simulink library "halin"  (R2021b)
settings: Solver=VariableStepAuto  StartTime=0.0  StopTime=10.0  RelTol=1e-3
undefined symbols (not defined in the file): TRUE
libraries: FVT_lib x177, hcu_lib x55
(part 4 of 17)

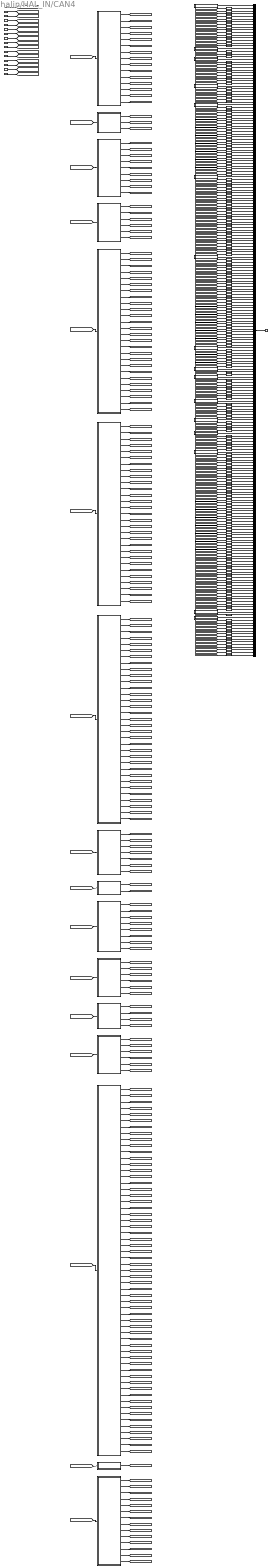
== system halin/HAL_IN/CAN4 ==
  DT_CAN4_SG_DKC1 : Inport
  DT_CAN4_SG_DKC2 : Inport  Port=2
  DT_CAN4_SG_PTG1 : Inport  Port=3
  DT_CAN4_SG_ZONE_DR1 : Inport  Port=4
  DT_CAN4_SG_ZONE_DR_VCU : Inport  Port=5
  DT_CAN4_SG_ZONE_FR1 : Inport  Port=6
  DT_CAN4_SG_ZONE_FR_VCU : Inport  Port=7
  DT_CAN4_SG_ZONE_L1 : Inport  Port=8
  DT_CAN4_SG_ZONE_L2 : Inport  Port=9
  DT_CAN4_SG_ZONE_R1 : Inport  Port=10
  DT_CAN4_SG_ZONE_R2 : Inport  Port=11
  DT_CAN4_SG_zGW_APTC1 : Inport  Port=12
  DT_CAN4_SG_zGW_CANFr1 : Inport  Port=13
  DT_CAN4_SG_zGW_LINDr1 : Inport  Port=14
  DT_CAN4_SG_zGW_LINFr1 : Inport  Port=15
  DT_CAN4_SG_zGW_SEAT1 : Inport  Port=16
  DKC1 : Subsystem
  DKC2 : Subsystem
  PTG1 : Subsystem
  UnitConverter{,1..11,13,18,21..22,24..26,33,39,41,43,45,47,49,51,53,55,57..58,82,88,90,92..97,100,102,104,106,108,110,112,114..118,120,124..127,131..134,137,140..143,155..156,158..160,165,169,173,177,180,213,218,220..221,224,226..227} (83 alike) : DataTypeConversion  OutDataTypeStr=uint8
  UnitConverter{29..30,38,40,42,44,46,48,50,52,54,56,61,63,84..87,89,91,99,101,103,105,107,109,111,113,119,128..129,138..139,144..152,164,168,172,176} (46 alike) : DataTypeConversion  OutDataTypeStr=single
  UnitConverter{12,14,19..20,23,27..28,31..32,34..37,59..60,62,64..81,83,98,121..123,130,135..136,154,157,161..163,166..167,170..171,174..175,178..179,181..212,214..216,222} (91 alike) : DataTypeConversion  OutDataTypeStr=boolean
  UnitConverter15 : DataTypeConversion  OutDataTypeStr=uint64
  UnitConverter{153,217,219,223,225} (5 alike) : DataTypeConversion  OutDataTypeStr=uint16
  UnitConverter16 : DataTypeConversion  OutDataTypeStr=uint64
  UnitConverter17 : DataTypeConversion  OutDataTypeStr=uint64
  VHAL_CANMsgInvalidDKC1_flg : Subsystem  AncestorBlock=FVT_lib/hal/MsgTimeoutJudge_CAN_AUTOSAR
      mask help: MeasumentTrigerEvent
      mask Display: fprintf('MsgTimeoutJudge_CAN\nAUTOSAR');
  VHAL_CANMsgInvalidDKC2_flg : Subsystem  AncestorBlock=FVT_lib/hal/MsgTimeoutJudge_CAN_AUTOSAR
      mask help: MeasumentTrigerEvent
      mask Display: fprintf('MsgTimeoutJudge_CAN\nAUTOSAR');
  VHAL_CANMsgInvalidPTG1_flg : Subsystem  AncestorBlock=FVT_lib/hal/MsgTimeoutJudge_CAN_AUTOSAR
      mask help: MeasumentTrigerEvent
      mask Display: fprintf('MsgTimeoutJudge_CAN\nAUTOSAR');
  VHAL_CANMsgInvalidZONEDR1_flg : Subsystem  AncestorBlock=FVT_lib/hal/MsgTimeoutJudge_CAN_AUTOSAR
      mask help: MeasumentTrigerEvent
      mask Display: fprintf('MsgTimeoutJudge_CAN\nAUTOSAR');
  VHAL_CANMsgInvalidZONEDRVCU_flg : Subsystem  AncestorBlock=FVT_lib/hal/MsgTimeoutJudge_CAN_AUTOSAR
      mask help: MeasumentTrigerEvent
      mask Display: fprintf('MsgTimeoutJudge_CAN\nAUTOSAR');
  VHAL_CANMsgInvalidZONEFR1_flg : Subsystem  AncestorBlock=FVT_lib/hal/MsgTimeoutJudge_CAN_AUTOSAR
      mask help: MeasumentTrigerEvent
      mask Display: fprintf('MsgTimeoutJudge_CAN\nAUTOSAR');
  VHAL_CANMsgInvalidZONEFRVCU_flg : Subsystem  AncestorBlock=FVT_lib/hal/MsgTimeoutJudge_CAN_AUTOSAR
      mask help: MeasumentTrigerEvent
      mask Display: fprintf('MsgTimeoutJudge_CAN\nAUTOSAR');
  VHAL_CANMsgInvalidZONEL1_flg : Subsystem  AncestorBlock=FVT_lib/hal/MsgTimeoutJudge_CAN_AUTOSAR
      mask help: MeasumentTrigerEvent
      mask Display: fprintf('MsgTimeoutJudge_CAN\nAUTOSAR');
  VHAL_CANMsgInvalidZONEL2_flg : Subsystem  AncestorBlock=FVT_lib/hal/MsgTimeoutJudge_CAN_AUTOSAR
      mask help: MeasumentTrigerEvent
      mask Display: fprintf('MsgTimeoutJudge_CAN\nAUTOSAR');
  VHAL_CANMsgInvalidZONER1_flg : Subsystem  AncestorBlock=FVT_lib/hal/MsgTimeoutJudge_CAN_AUTOSAR
      mask help: MeasumentTrigerEvent
      mask Display: fprintf('MsgTimeoutJudge_CAN\nAUTOSAR');
  VHAL_CANMsgInvalidZONER2_flg : Subsystem  AncestorBlock=FVT_lib/hal/MsgTimeoutJudge_CAN_AUTOSAR
      mask help: MeasumentTrigerEvent
      mask Display: fprintf('MsgTimeoutJudge_CAN\nAUTOSAR');
  VHAL_CANMsgInvalidzGWAPTC1_flg : Subsystem  AncestorBlock=FVT_lib/hal/MsgTimeoutJudge_CAN_AUTOSAR
      mask help: MeasumentTrigerEvent
      mask Display: fprintf('MsgTimeoutJudge_CAN\nAUTOSAR');
  VHAL_CANMsgInvalidzGWCANFr1_flg : Subsystem  AncestorBlock=FVT_lib/hal/MsgTimeoutJudge_CAN_AUTOSAR
      mask help: MeasumentTrigerEvent
      mask Display: fprintf('MsgTimeoutJudge_CAN\nAUTOSAR');
  VHAL_CANMsgInvalidzGWLINDr1_flg : Subsystem  AncestorBlock=FVT_lib/hal/MsgTimeoutJudge_CAN_AUTOSAR
      mask help: MeasumentTrigerEvent
      mask Display: fprintf('MsgTimeoutJudge_CAN\nAUTOSAR');
  VHAL_CANMsgInvalidzGWLINFr1_flg : Subsystem  AncestorBlock=FVT_lib/hal/MsgTimeoutJudge_CAN_AUTOSAR
      mask help: MeasumentTrigerEvent
      mask Display: fprintf('MsgTimeoutJudge_CAN\nAUTOSAR');
  VHAL_CANMsgInvalidzGWSEAT1_flg : Subsystem  AncestorBlock=FVT_lib/hal/MsgTimeoutJudge_CAN_AUTOSAR
      mask help: MeasumentTrigerEvent
      mask Display: fprintf('MsgTimeoutJudge_CAN\nAUTOSAR');
  ZONE_DR1 : Subsystem
  ZONE_DR_VCU : Subsystem
  ZONE_FR1 : Subsystem
  ZONE_FR_VCU : Subsystem
  ZONE_L1 : Subsystem
  ZONE_L2 : Subsystem
  ZONE_R1 : Subsystem
  ZONE_R2 : Subsystem
  bus_creator : BusCreator  Inputs=244
  zGW_APTC1 : Subsystem
  zGW_CANFr1 : Subsystem
  zGW_LINDr1 : Subsystem
  zGW_LINFr1 : Subsystem
  zGW_SEAT1 : Subsystem
  HAL_CAN4_outputs : Outport
  wires:
  DT_CAN4_SG_DKC1/1 -> [DT_CAN4_SG_DKC1]
  DT_CAN4_SG_DKC2/1 -> [DT_CAN4_SG_DKC2]
  DT_CAN4_SG_PTG1/1 -> [DT_CAN4_SG_PTG1]
  DT_CAN4_SG_ZONE_DR1/1 -> [DT_CAN4_SG_ZONE_DR1]
  DT_CAN4_SG_ZONE_DR_VCU/1 -> [DT_CAN4_SG_ZONE_DR_VCU]
  DT_CAN4_SG_ZONE_FR1/1 -> [DT_CAN4_SG_ZONE_FR1]
  DT_CAN4_SG_ZONE_FR_VCU/1 -> [DT_CAN4_SG_ZONE_FR_VCU]
  DT_CAN4_SG_ZONE_L1/1 -> [DT_CAN4_SG_ZONE_L1]
  DT_CAN4_SG_ZONE_L2/1 -> [DT_CAN4_SG_ZONE_L2]
  DT_CAN4_SG_ZONE_R1/1 -> [DT_CAN4_SG_ZONE_R1]
  DT_CAN4_SG_ZONE_R2/1 -> [DT_CAN4_SG_ZONE_R2]
  DT_CAN4_SG_zGW_APTC1/1 -> [DT_CAN4_SG_zGW_APTC1]
  DT_CAN4_SG_zGW_CANFr1/1 -> [DT_CAN4_SG_zGW_CANFr1]
  DT_CAN4_SG_zGW_LINDr1/1 -> [DT_CAN4_SG_zGW_LINDr1]
  DT_CAN4_SG_zGW_LINFr1/1 -> [DT_CAN4_SG_zGW_LINFr1]
  DT_CAN4_SG_zGW_SEAT1/1 -> [DT_CAN4_SG_zGW_SEAT1]
  [DT_CAN4_SG_DKC1] -> DKC1/1(DT_CAN4_SG_DKC1)
  [DT_CAN4_SG_DKC2] -> DKC2/1(DT_CAN4_SG_DKC2)
  [DT_CAN4_SG_PTG1] -> PTG1/1(DT_CAN4_SG_PTG1)
  [DT_CAN4_SG_ZONE_DR1] -> ZONE_DR1/1(DT_CAN4_SG_ZONE_DR1)
  [DT_CAN4_SG_ZONE_DR_VCU] -> ZONE_DR_VCU/1(DT_CAN4_SG_ZONE_DR_VCU)
  [DT_CAN4_SG_ZONE_FR1] -> ZONE_FR1/1(DT_CAN4_SG_ZONE_FR1)
  [DT_CAN4_SG_ZONE_FR_VCU] -> ZONE_FR_VCU/1(DT_CAN4_SG_ZONE_FR_VCU)
  [DT_CAN4_SG_ZONE_L1] -> ZONE_L1/1(DT_CAN4_SG_ZONE_L1)
  [DT_CAN4_SG_ZONE_L2] -> ZONE_L2/1(DT_CAN4_SG_ZONE_L2)
  [DT_CAN4_SG_ZONE_R1] -> ZONE_R1/1(DT_CAN4_SG_ZONE_R1)
  [DT_CAN4_SG_ZONE_R2] -> ZONE_R2/1(DT_CAN4_SG_ZONE_R2)
  [DT_CAN4_SG_zGW_APTC1] -> zGW_APTC1/1(DT_CAN4_SG_zGW_APTC1)
  [DT_CAN4_SG_zGW_CANFr1] -> zGW_CANFr1/1(DT_CAN4_SG_zGW_CANFr1)
  [DT_CAN4_SG_zGW_LINDr1] -> zGW_LINDr1/1(DT_CAN4_SG_zGW_LINDr1)
  [DT_CAN4_SG_zGW_LINFr1] -> zGW_LINFr1/1(DT_CAN4_SG_zGW_LINFr1)
  [DT_CAN4_SG_zGW_SEAT1] -> zGW_SEAT1/1(DT_CAN4_SG_zGW_SEAT1)
  bus_creator/1 -> HAL_CAN4_outputs/1
  VHAL_CANMsgInvalidDKC1_flg/1(Out) -> bus_creator/1
  DKC1/1(VHAL_DKCKeyNumSta_enum) -> [VHAL_DKCKeyNumSta_enum]
  UnitConverter/1 -> bus_creator/2  "VHAL_DKCKeyNumSta_enum"
  [VHAL_DKCKeyNumSta_enum] -> UnitConverter/1
  DKC1/2(VHAL_DKCKeyTypeSta_enum) -> [VHAL_DKCKeyTypeSta_enum]
  UnitConverter1/1 -> bus_creator/3  "VHAL_DKCKeyTypeSta_enum"
  [VHAL_DKCKeyTypeSta_enum] -> UnitConverter1/1
  DKC1/3(VHAL_DKCPDkeyAreaRAPSSta_enum) -> [VHAL_DKCPDkeyAreaRAPSSta_enum]
  UnitConverter2/1 -> bus_creator/4  "VHAL_DKCPDkeyAreaRAPSSta_enum"
  [VHAL_DKCPDkeyAreaRAPSSta_enum] -> UnitConverter2/1
  DKC1/4(VHAL_DKCParkingModeCmd_enum) -> [VHAL_DKCParkingModeCmd_enum]
  UnitConverter3/1 -> bus_creator/5  "VHAL_DKCParkingModeCmd_enum"
  [VHAL_DKCParkingModeCmd_enum] -> UnitConverter3/1
  DKC1/5(VHAL_DKCReVehData_enum) -> [VHAL_DKCReVehData_enum]
  UnitConverter4/1 -> bus_creator/6  "VHAL_DKCReVehData_enum"
  [VHAL_DKCReVehData_enum] -> UnitConverter4/1
  DKC1/6(VHAL_PCommandToBCM_enum) -> [VHAL_PCommandToBCM_enum]
  UnitConverter5/1 -> bus_creator/7  "VHAL_PCommandToBCM_enum"
  [VHAL_PCommandToBCM_enum] -> UnitConverter5/1
  DKC1/7(VHAL_PCommandToPTG_enum) -> [VHAL_PCommandToPTG_enum]
  UnitConverter6/1 -> bus_creator/8  "VHAL_PCommandToPTG_enum"
  [VHAL_PCommandToPTG_enum] -> UnitConverter6/1
  DKC1/8(VHAL_PDKeyAreaLockUnlock_enum) -> [VHAL_PDKeyAreaLockUnlock_enum]
  UnitConverter7/1 -> bus_creator/9  "VHAL_PDKeyAreaLockUnlock_enum"
  [VHAL_PDKeyAreaLockUnlock_enum] -> UnitConverter7/1
  DKC1/9(VHAL_PDKeyAreaPS_enum) -> [VHAL_PDKeyAreaPS_enum]
  UnitConverter8/1 -> bus_creator/10  "VHAL_PDKeyAreaPS_enum"
  [VHAL_PDKeyAreaPS_enum] -> UnitConverter8/1
  DKC1/10(VHAL_PDKeyAreaPTG_enum) -> [VHAL_PDKeyAreaPTG_enum]
  UnitConverter9/1 -> bus_creator/11  "VHAL_PDKeyAreaPTG_enum"
  [VHAL_PDKeyAreaPTG_enum] -> UnitConverter9/1
  DKC1/11(VHAL_PDKeyWelcome_enum) -> [VHAL_PDKeyWelcome_enum]
  UnitConverter10/1 -> bus_creator/12  "VHAL_PDKeyWelcome_enum"
  [VHAL_PDKeyWelcome_enum] -> UnitConverter10/1
  DKC1/12(VHAL_PDkeyShowIVI_enum) -> [VHAL_PDkeyShowIVI_enum]
  UnitConverter11/1 -> bus_creator/13  "VHAL_PDkeyShowIVI_enum"
  [VHAL_PDkeyShowIVI_enum] -> UnitConverter11/1
  DKC1/13(VHAL_PKeyMiss_flg) -> [VHAL_PKeyMiss_flg]
  UnitConverter12/1 -> bus_creator/14  "VHAL_PKeyMiss_flg"
  [VHAL_PKeyMiss_flg] -> UnitConverter12/1
  DKC1/14(VHAL_PKeyMode_enum) -> [VHAL_PKeyMode_enum]
  UnitConverter13/1 -> bus_creator/15  "VHAL_PKeyMode_enum"
  [VHAL_PKeyMode_enum] -> UnitConverter13/1
  DKC1/15(VHAL_PUIDLowPower_flg) -> [VHAL_PUIDLowPower_flg]
  UnitConverter14/1 -> bus_creator/16  "VHAL_PUIDLowPower_flg"
  [VHAL_PUIDLowPower_flg] -> UnitConverter14/1
  VHAL_CANMsgInvalidDKC2_flg/1(Out) -> bus_creator/17
  DKC2/1(VHAL_EncryptionDATA063_enum) -> [VHAL_EncryptionDATA063_enum]
  UnitConverter15/1 -> bus_creator/18  "VHAL_EncryptionDATA063_enum"
  [VHAL_EncryptionDATA063_enum] -> UnitConverter15/1
  DKC2/2(VHAL_EncryptionDATA64127_enum) -> [VHAL_EncryptionDATA64127_enum]
  UnitConverter16/1 -> bus_creator/19  "VHAL_EncryptionDATA64127_enum"
  [VHAL_EncryptionDATA64127_enum] -> UnitConverter16/1
  DKC2/3(VHAL_RandomNumberX_enum) -> [VHAL_RandomNumberX_enum]
  UnitConverter17/1 -> bus_creator/20  "VHAL_RandomNumberX_enum"
  [VHAL_RandomNumberX_enum] -> UnitConverter17/1
  VHAL_CANMsgInvalidPTG1_flg/1(Out) -> bus_creator/21
  PTG1/1(VHAL_PTGActiveSta_enum) -> [VHAL_PTGActiveSta_enum]
  UnitConverter18/1 -> bus_creator/22  "VHAL_PTGActiveSta_enum"
  [VHAL_PTGActiveSta_enum] -> UnitConverter18/1
  PTG1/2(VHAL_PTGAutoStaus_flg) -> [VHAL_PTGAutoStaus_flg]
  UnitConverter19/1 -> bus_creator/23  "VHAL_PTGAutoStaus_flg"
  [VHAL_PTGAutoStaus_flg] -> UnitConverter19/1
  PTG1/3(VHAL_PTGExist_flg) -> [VHAL_PTGExist_flg]
  UnitConverter20/1 -> bus_creator/24  "VHAL_PTGExist_flg"
  [VHAL_PTGExist_flg] -> UnitConverter20/1
  PTG1/4(VHAL_PTGHWVer_enum) -> [VHAL_PTGHWVer_enum]
  UnitConverter21/1 -> bus_creator/25  "VHAL_PTGHWVer_enum"
  [VHAL_PTGHWVer_enum] -> UnitConverter21/1
  PTG1/5(VHAL_PTGInnerSW2_enum) -> [VHAL_PTGInnerSW2_enum]
  UnitConverter22/1 -> bus_creator/26  "VHAL_PTGInnerSW2_enum"
  [VHAL_PTGInnerSW2_enum] -> UnitConverter22/1
  PTG1/6(VHAL_PTGIsSetHeight_flg) -> [VHAL_PTGIsSetHeight_flg]
  UnitConverter23/1 -> bus_creator/27  "VHAL_PTGIsSetHeight_flg"
  [VHAL_PTGIsSetHeight_flg] -> UnitConverter23/1
  PTG1/7(VHAL_PTGRDILSta_enum) -> [VHAL_PTGRDILSta_enum]
  UnitConverter24/1 -> bus_creator/28  "VHAL_PTGRDILSta_enum"
  [VHAL_PTGRDILSta_enum] -> UnitConverter24/1
  PTG1/8(VHAL_PTGSWVer_enum) -> [VHAL_PTGSWVer_enum]
  UnitConverter25/1 -> bus_creator/29  "VHAL_PTGSWVer_enum"
  [VHAL_PTGSWVer_enum] -> UnitConverter25/1
  PTG1/9(VHAL_PTGSysSta_enum) -> [VHAL_PTGSysSta_enum]
  UnitConverter26/1 -> bus_creator/30  "VHAL_PTGSysSta_enum"
  [VHAL_PTGSysSta_enum] -> UnitConverter26/1
  VHAL_CANMsgInvalidZONEDR1_flg/1(Out) -> bus_creator/31
  ZONE_DR1/1(VHAL_DrLockSta_flg) -> [VHAL_DrLockSta_flg]
  UnitConverter27/1 -> bus_creator/32  "VHAL_DrLockSta_flg"
  [VHAL_DrLockSta_flg] -> UnitConverter27/1
  ZONE_DR1/2(VHAL_MIRRORFOLDSW_flg) -> [VHAL_MIRRORFOLDSW_flg]
  UnitConverter28/1 -> bus_creator/33  "VHAL_MIRRORFOLDSW_flg"
  [VHAL_MIRRORFOLDSW_flg] -> UnitConverter28/1
  ZONE_DR1/3(VHAL_RLTurnLampC_mA) -> [VHAL_RLTurnLampC_mA]
  UnitConverter29/1 -> bus_creator/34  "VHAL_RLTurnLampC_mA"
  [VHAL_RLTurnLampC_mA] -> UnitConverter29/1
  ZONE_DR1/4(VHAL_RRTurnLampC_mA) -> [VHAL_RRTurnLampC_mA]
  UnitConverter30/1 -> bus_creator/35  "VHAL_RRTurnLampC_mA"
  [VHAL_RRTurnLampC_mA] -> UnitConverter30/1
  ZONE_DR1/5(VHAL_RWiperAS_flg) -> [VHAL_RWiperAS_flg]
  UnitConverter31/1 -> bus_creator/36  "VHAL_RWiperAS_flg"
  [VHAL_RWiperAS_flg] -> UnitConverter31/1
  ZONE_DR1/6(VHAL_RWiperProtection_flg) -> [VHAL_RWiperProtection_flg]
  UnitConverter32/1 -> bus_creator/37  "VHAL_RWiperProtection_flg"
  [VHAL_RWiperProtection_flg] -> UnitConverter32/1
  VHAL_CANMsgInvalidZONEDRVCU_flg/1(Out) -> bus_creator/38
  ZONE_DR_VCU/1(VHAL_BlowerErr_enum) -> [VHAL_BlowerErr_enum]
  UnitConverter33/1 -> bus_creator/39  "VHAL_BlowerErr_enum"
  [VHAL_BlowerErr_enum] -> UnitConverter33/1
  ZONE_DR_VCU/2(VHAL_DrPMMLVOutPErrLmp_flg) -> [VHAL_DrPMMLVOutPErrLmp_flg]
  UnitConverter34/1 -> bus_creator/40  "VHAL_DrPMMLVOutPErrLmp_flg"
  [VHAL_DrPMMLVOutPErrLmp_flg] -> UnitConverter34/1
  ZONE_DR_VCU/3(VHAL_DrPMMSysErrLmp_flg) -> [VHAL_DrPMMSysErrLmp_flg]
  UnitConverter35/1 -> bus_creator/41  "VHAL_DrPMMSysErrLmp_flg"
  [VHAL_DrPMMSysErrLmp_flg] -> UnitConverter35/1
  ZONE_DR_VCU/4(VHAL_DrSCPSysErrLmp_flg) -> [VHAL_DrSCPSysErrLmp_flg]
  UnitConverter36/1 -> bus_creator/42  "VHAL_DrSCPSysErrLmp_flg"
  [VHAL_DrSCPSysErrLmp_flg] -> UnitConverter36/1
  ZONE_DR_VCU/5(VHAL_DrStdAErrSta_flg) -> [VHAL_DrStdAErrSta_flg]
  UnitConverter37/1 -> bus_creator/43  "VHAL_DrStdAErrSta_flg"
  [VHAL_DrStdAErrSta_flg] -> UnitConverter37/1
  ZONE_DR_VCU/6(VHAL_SolarL_W) -> [VHAL_SolarL_W]
  UnitConverter38/1 -> bus_creator/44  "VHAL_SolarL_W"
  [VHAL_SolarL_W] -> UnitConverter38/1
  ZONE_DR_VCU/7(VHAL_SolarLErr_enum) -> [VHAL_SolarLErr_enum]
  UnitConverter39/1 -> bus_creator/45  "VHAL_SolarLErr_enum"
  [VHAL_SolarLErr_enum] -> UnitConverter39/1
  ZONE_DR_VCU/8(VHAL_SolarR_W) -> [VHAL_SolarR_W]
  UnitConverter40/1 -> bus_creator/46  "VHAL_SolarR_W"
  [VHAL_SolarR_W] -> UnitConverter40/1
  ZONE_DR_VCU/9(VHAL_SolarRErr_enum) -> [VHAL_SolarRErr_enum]
  UnitConverter41/1 -> bus_creator/47  "VHAL_SolarRErr_enum"
  [VHAL_SolarRErr_enum] -> UnitConverter41/1
  ZONE_DR_VCU/10(VHAL_TFaceL_C) -> [VHAL_TFaceL_C]
  UnitConverter42/1 -> bus_creator/48  "VHAL_TFaceL_C"
  [VHAL_TFaceL_C] -> UnitConverter42/1
  ZONE_DR_VCU/11(VHAL_TFaceLErr_enum) -> [VHAL_TFaceLErr_enum]
  UnitConverter43/1 -> bus_creator/49  "VHAL_TFaceLErr_enum"
  [VHAL_TFaceLErr_enum] -> UnitConverter43/1
  ZONE_DR_VCU/12(VHAL_TFaceR_C) -> [VHAL_TFaceR_C]
  UnitConverter44/1 -> bus_creator/50  "VHAL_TFaceR_C"
  [VHAL_TFaceR_C] -> UnitConverter44/1
  ZONE_DR_VCU/13(VHAL_TFaceRErr_enum) -> [VHAL_TFaceRErr_enum]
  UnitConverter45/1 -> bus_creator/51  "VHAL_TFaceRErr_enum"
  [VHAL_TFaceRErr_enum] -> UnitConverter45/1
  ZONE_DR_VCU/14(VHAL_TFaceRr_C) -> [VHAL_TFaceRr_C]
  UnitConverter46/1 -> bus_creator/52  "VHAL_TFaceRr_C"
  [VHAL_TFaceRr_C] -> UnitConverter46/1
  ZONE_DR_VCU/15(VHAL_TFaceRrErr_enum) -> [VHAL_TFaceRrErr_enum]
  UnitConverter47/1 -> bus_creator/53  "VHAL_TFaceRrErr_enum"
  [VHAL_TFaceRrErr_enum] -> UnitConverter47/1
  ZONE_DR_VCU/16(VHAL_TFootL_C) -> [VHAL_TFootL_C]
  UnitConverter48/1 -> bus_creator/54  "VHAL_TFootL_C"
  [VHAL_TFootL_C] -> UnitConverter48/1
  ZONE_DR_VCU/17(VHAL_TFootLErr_enum) -> [VHAL_TFootLErr_enum]
  UnitConverter49/1 -> bus_creator/55  "VHAL_TFootLErr_enum"
  [VHAL_TFootLErr_enum] -> UnitConverter49/1
  ZONE_DR_VCU/18(VHAL_TFootR_C) -> [VHAL_TFootR_C]
  UnitConverter50/1 -> bus_creator/56  "VHAL_TFootR_C"
  [VHAL_TFootR_C] -> UnitConverter50/1
  ZONE_DR_VCU/19(VHAL_TFootRErr_enum) -> [VHAL_TFootRErr_enum]
  UnitConverter51/1 -> bus_creator/57  "VHAL_TFootRErr_enum"
  [VHAL_TFootRErr_enum] -> UnitConverter51/1
  ZONE_DR_VCU/20(VHAL_TFootRr_C) -> [VHAL_TFootRr_C]
  UnitConverter52/1 -> bus_creator/58  "VHAL_TFootRr_C"
  [VHAL_TFootRr_C] -> UnitConverter52/1
  ZONE_DR_VCU/21(VHAL_TFootRrErr_enum) -> [VHAL_TFootRrErr_enum]
  UnitConverter53/1 -> bus_creator/59  "VHAL_TFootRrErr_enum"
  [VHAL_TFootRrErr_enum] -> UnitConverter53/1
  ZONE_DR_VCU/22(VHAL_Tevap_C) -> [VHAL_Tevap_C]
  UnitConverter54/1 -> bus_creator/60  "VHAL_Tevap_C"
  [VHAL_Tevap_C] -> UnitConverter54/1
  ZONE_DR_VCU/23(VHAL_TevapErr_enum) -> [VHAL_TevapErr_enum]
  UnitConverter55/1 -> bus_creator/61  "VHAL_TevapErr_enum"
  [VHAL_TevapErr_enum] -> UnitConverter55/1
  ZONE_DR_VCU/24(VHAL_Tincar_C) -> [VHAL_Tincar_C]
  UnitConverter56/1 -> bus_creator/62  "VHAL_Tincar_C"
  [VHAL_Tincar_C] -> UnitConverter56/1
  ZONE_DR_VCU/25(VHAL_TincarErr_enum) -> [VHAL_TincarErr_enum]
  UnitConverter57/1 -> bus_creator/63  "VHAL_TincarErr_enum"
  [VHAL_TincarErr_enum] -> UnitConverter57/1
  ZONE_DR_VCU/26(VHAL_ZoneDrMalfunLevel_enum) -> [VHAL_ZoneDrMalfunLevel_enum]
  UnitConverter58/1 -> bus_creator/64  "VHAL_ZoneDrMalfunLevel_enum"
  [VHAL_ZoneDrMalfunLevel_enum] -> UnitConverter58/1
  VHAL_CANMsgInvalidZONEFR1_flg/1(Out) -> bus_creator/65
  ZONE_FR1/1(VHAL_ChargeInletLockSta_flg) -> [VHAL_ChargeInletLockSta_flg]
  UnitConverter59/1 -> bus_creator/66  "VHAL_ChargeInletLockSta_flg"
  [VHAL_ChargeInletLockSta_flg] -> UnitConverter59/1
  ZONE_FR1/2(VHAL_CompProEN_flg) -> [VHAL_CompProEN_flg]
  UnitConverter60/1 -> bus_creator/67  "VHAL_CompProEN_flg"
  [VHAL_CompProEN_flg] -> UnitConverter60/1
  ZONE_FR1/3(VHAL_FLTurnLampC_mA) -> [VHAL_FLTurnLampC_mA]
  UnitConverter61/1 -> bus_creator/68  "VHAL_FLTurnLampC_mA"
  [VHAL_FLTurnLampC_mA] -> UnitConverter61/1
  ZONE_FR1/4(VHAL_FLTurnLightWarning_flg) -> [VHAL_FLTurnLightWarning_flg]
  UnitConverter62/1 -> bus_creator/69  "VHAL_FLTurnLightWarning_flg"
  [VHAL_FLTurnLightWarning_flg] -> UnitConverter62/1
  ZONE_FR1/5(VHAL_FRTurnLampC_mA) -> [VHAL_FRTurnLampC_mA]
  UnitConverter63/1 -> bus_creator/70  "VHAL_FRTurnLampC_mA"
  [VHAL_FRTurnLampC_mA] -> UnitConverter63/1
  ZONE_FR1/6(VHAL_FRTurnLightWarning_flg) -> [VHAL_FRTurnLightWarning_flg]
  UnitConverter64/1 -> bus_creator/71  "VHAL_FRTurnLightWarning_flg"
  [VHAL_FRTurnLightWarning_flg] -> UnitConverter64/1
  ZONE_FR1/7(VHAL_FWiperAS_flg) -> [VHAL_FWiperAS_flg]
  UnitConverter65/1 -> bus_creator/72  "VHAL_FWiperAS_flg"
  [VHAL_FWiperAS_flg] -> UnitConverter65/1
  ZONE_FR1/8(VHAL_FWiperProtection_flg) -> [VHAL_FWiperProtection_flg]
  UnitConverter66/1 -> bus_creator/73  "VHAL_FWiperProtection_flg"
  [VHAL_FWiperProtection_flg] -> UnitConverter66/1
  ZONE_FR1/9(VHAL_LADBHibeamIndication_flg) -> [VHAL_LADBHibeamIndication_flg]
  UnitConverter67/1 -> bus_creator/74  "VHAL_LADBHibeamIndication_flg"
  [VHAL_LADBHibeamIndication_flg] -> UnitConverter67/1
  ZONE_FR1/10(VHAL_LADBOperationStatus_flg) -> [VHAL_LADBOperationStatus_flg]
  UnitConverter68/1 -> bus_creator/75  "VHAL_LADBOperationStatus_flg"
  [VHAL_LADBOperationStatus_flg] -> UnitConverter68/1
  ZONE_FR1/11(VHAL_LADBWarning_flg) -> [VHAL_LADBWarning_flg]
  UnitConverter69/1 -> bus_creator/76  "VHAL_LADBWarning_flg"
  [VHAL_LADBWarning_flg] -> UnitConverter69/1
  ZONE_FR1/12(VHAL_LAHBWarning_flg) -> [VHAL_LAHBWarning_flg]
  UnitConverter70/1 -> bus_creator/77  "VHAL_LAHBWarning_flg"
  [VHAL_LAHBWarning_flg] -> UnitConverter70/1
  ZONE_FR1/13(VHAL_LDRLWarning_flg) -> [VHAL_LDRLWarning_flg]
  UnitConverter71/1 -> bus_creator/78  "VHAL_LDRLWarning_flg"
  [VHAL_LDRLWarning_flg] -> UnitConverter71/1
  ZONE_FR1/14(VHAL_LLBWarning_flg) -> [VHAL_LLBWarning_flg]
  UnitConverter72/1 -> bus_creator/79  "VHAL_LLBWarning_flg"
  [VHAL_LLBWarning_flg] -> UnitConverter72/1
  ZONE_FR1/15(VHAL_LpositionLampWarning_flg) -> [VHAL_LpositionLampWarning_flg]
  UnitConverter73/1 -> bus_creator/80  "VHAL_LpositionLampWarning_flg"
  [VHAL_LpositionLampWarning_flg] -> UnitConverter73/1
  ZONE_FR1/16(VHAL_RADBHibeamIndication_flg) -> [VHAL_RADBHibeamIndication_flg]
  UnitConverter74/1 -> bus_creator/81  "VHAL_RADBHibeamIndication_flg"
  [VHAL_RADBHibeamIndication_flg] -> UnitConverter74/1
  ZONE_FR1/17(VHAL_RADBOperationStatus_flg) -> [VHAL_RADBOperationStatus_flg]
  UnitConverter75/1 -> bus_creator/82  "VHAL_RADBOperationStatus_flg"
  [VHAL_RADBOperationStatus_flg] -> UnitConverter75/1
  ZONE_FR1/18(VHAL_RADBWarning_flg) -> [VHAL_RADBWarning_flg]
  UnitConverter76/1 -> bus_creator/83  "VHAL_RADBWarning_flg"
  [VHAL_RADBWarning_flg] -> UnitConverter76/1
  ZONE_FR1/19(VHAL_RAHBWarning_flg) -> [VHAL_RAHBWarning_flg]
  UnitConverter77/1 -> bus_creator/84  "VHAL_RAHBWarning_flg"
  [VHAL_RAHBWarning_flg] -> UnitConverter77/1
  ZONE_FR1/20(VHAL_RDRLWarning_flg) -> [VHAL_RDRLWarning_flg]
  UnitConverter78/1 -> bus_creator/85  "VHAL_RDRLWarning_flg"
  [VHAL_RDRLWarning_flg] -> UnitConverter78/1
  ZONE_FR1/21(VHAL_RLBWarning_flg) -> [VHAL_RLBWarning_flg]
  UnitConverter79/1 -> bus_creator/86  "VHAL_RLBWarning_flg"
  [VHAL_RLBWarning_flg] -> UnitConverter79/1
  ZONE_FR1/22(VHAL_RpositionLampWarning_flg) -> [VHAL_RpositionLampWarning_flg]
  UnitConverter80/1 -> bus_creator/87  "VHAL_RpositionLampWarning_flg"
  [VHAL_RpositionLampWarning_flg] -> UnitConverter80/1
  ZONE_FR1/23(VHAL_TrailerCheck_flg) -> [VHAL_TrailerCheck_flg]
  UnitConverter81/1 -> bus_creator/88  "VHAL_TrailerCheck_flg"
  [VHAL_TrailerCheck_flg] -> UnitConverter81/1
  ZONE_FR1/24(VHAL_TrailerModeSta_enum) -> [VHAL_TrailerModeSta_enum]
  UnitConverter82/1 -> bus_creator/89  "VHAL_TrailerModeSta_enum"
  [VHAL_TrailerModeSta_enum] -> UnitConverter82/1
  ZONE_FR1/25(VHAL_ZFRBCMChargerDoorSWSta_flg) -> [VHAL_ZFRBCMChargerDoorSWSta_flg]
  UnitConverter83/1 -> bus_creator/90  "VHAL_ZFRBCMChargerDoorSWSta_flg"
  [VHAL_ZFRBCMChargerDoorSWSta_flg] -> UnitConverter83/1
  ZONE_FR1/26(VHAL_ZFRTHCMCLEVentActYSta_pct) -> [VHAL_ZFRTHCMCLEVentActYSta_pct]
  UnitConverter84/1 -> bus_creator/91  "VHAL_ZFRTHCMCLEVentActYSta_pct"
  [VHAL_ZFRTHCMCLEVentActYSta_pct] -> UnitConverter84/1
  ZONE_FR1/27(VHAL_ZFRTHCMCREVentActYSta_pct) -> [VHAL_ZFRTHCMCREVentActYSta_pct]
  UnitConverter85/1 -> bus_creator/92  "VHAL_ZFRTHCMCREVentActYSta_pct"
  [VHAL_ZFRTHCMCREVentActYSta_pct] -> UnitConverter85/1
  ZONE_FR1/28(VHAL_ZFRTHCMDrEVentActYSta_pct) -> [VHAL_ZFRTHCMDrEVentActYSta_pct]
  UnitConverter86/1 -> bus_creator/93  "VHAL_ZFRTHCMDrEVentActYSta_pct"
  [VHAL_ZFRTHCMDrEVentActYSta_pct] -> UnitConverter86/1
  ZONE_FR1/29(VHAL_ZFRTHCMPsEVentActYSta_pct) -> [VHAL_ZFRTHCMPsEVentActYSta_pct]
  UnitConverter87/1 -> bus_creator/94  "VHAL_ZFRTHCMPsEVentActYSta_pct"
  [VHAL_ZFRTHCMPsEVentActYSta_pct] -> UnitConverter87/1
  VHAL_CANMsgInvalidZONEFRVCU_flg/1(Out) -> bus_creator/95
  ZONE_FR_VCU/1(VHAL_AGSErr_enum) -> [VHAL_AGSErr_enum]
  UnitConverter88/1 -> bus_creator/96  "VHAL_AGSErr_enum"
  [VHAL_AGSErr_enum] -> UnitConverter88/1
  ZONE_FR_VCU/2(VHAL_BatInTemp_C) -> [VHAL_BatInTemp_C]
  UnitConverter89/1 -> bus_creator/97  "VHAL_BatInTemp_C"
  [VHAL_BatInTemp_C] -> UnitConverter89/1
  ZONE_FR_VCU/3(VHAL_BatInTempErr_enum) -> [VHAL_BatInTempErr_enum]
  UnitConverter90/1 -> bus_creator/98  "VHAL_BatInTempErr_enum"
  [VHAL_BatInTempErr_enum] -> UnitConverter90/1
  ZONE_FR_VCU/4(VHAL_BatOutTemp_C) -> [VHAL_BatOutTemp_C]
  UnitConverter91/1 -> bus_creator/99  "VHAL_BatOutTemp_C"
  [VHAL_BatOutTemp_C] -> UnitConverter91/1
  ZONE_FR_VCU/5(VHAL_COMPErr_enum) -> [VHAL_COMPErr_enum]
  UnitConverter92/1 -> bus_creator/100  "VHAL_COMPErr_enum"
  [VHAL_COMPErr_enum] -> UnitConverter92/1
  ZONE_FR_VCU/6(VHAL_EACProtectEnable_enum) -> [VHAL_EACProtectEnable_enum]
  UnitConverter93/1 -> bus_creator/101  "VHAL_EACProtectEnable_enum"
  [VHAL_EACProtectEnable_enum] -> UnitConverter93/1
  ZONE_FR_VCU/7(VHAL_EWP3Err_enum) -> [VHAL_EWP3Err_enum]
  UnitConverter94/1 -> bus_creator/102  "VHAL_EWP3Err_enum"
  [VHAL_EWP3Err_enum] -> UnitConverter94/1
  ZONE_FR_VCU/8(VHAL_EXV1Err_enum) -> [VHAL_EXV1Err_enum]
  UnitConverter95/1 -> bus_creator/103  "VHAL_EXV1Err_enum"
  [VHAL_EXV1Err_enum] -> UnitConverter95/1
  ZONE_FR_VCU/9(VHAL_EXV2Err_enum) -> [VHAL_EXV2Err_enum]
  UnitConverter96/1 -> bus_creator/104  "VHAL_EXV2Err_enum"
  [VHAL_EXV2Err_enum] -> UnitConverter96/1
  ZONE_FR_VCU/10(VHAL_FanErr_enum) -> [VHAL_FanErr_enum]
  UnitConverter97/1 -> bus_creator/105  "VHAL_FanErr_enum"
  [VHAL_FanErr_enum] -> UnitConverter97/1
  ZONE_FR_VCU/11(VHAL_FrPMMLimpHomeActReq_flg) -> [VHAL_FrPMMLimpHomeActReq_flg]
  UnitConverter98/1 -> bus_creator/106  "VHAL_FrPMMLimpHomeActReq_flg"
  [VHAL_FrPMMLimpHomeActReq_flg] -> UnitConverter98/1
  ZONE_FR_VCU/12(VHAL_MotorInTemp_C) -> [VHAL_MotorInTemp_C]
  UnitConverter99/1 -> bus_creator/107  "VHAL_MotorInTemp_C"
  [VHAL_MotorInTemp_C] -> UnitConverter99/1
  ZONE_FR_VCU/13(VHAL_MotorInTempErr_enum) -> [VHAL_MotorInTempErr_enum]
  UnitConverter100/1 -> bus_creator/108  "VHAL_MotorInTempErr_enum"
  [VHAL_MotorInTempErr_enum] -> UnitConverter100/1
  ZONE_FR_VCU/14(VHAL_MotorOutTemp_C) -> [VHAL_MotorOutTemp_C]
  UnitConverter101/1 -> bus_creator/109  "VHAL_MotorOutTemp_C"
  [VHAL_MotorOutTemp_C] -> UnitConverter101/1
  ZONE_FR_VCU/15(VHAL_MotorOutTempErr_enum) -> [VHAL_MotorOutTempErr_enum]
  UnitConverter102/1 -> bus_creator/110  "VHAL_MotorOutTempErr_enum"
  [VHAL_MotorOutTempErr_enum] -> UnitConverter102/1
  ZONE_FR_VCU/16(VHAL_PTHighP_KPa) -> [VHAL_PTHighP_KPa]
  UnitConverter103/1 -> bus_creator/111  "VHAL_PTHighP_KPa"
  [VHAL_PTHighP_KPa] -> UnitConverter103/1
  ZONE_FR_VCU/17(VHAL_PTHighPErr_enum) -> [VHAL_PTHighPErr_enum]
  UnitConverter104/1 -> bus_creator/112  "VHAL_PTHighPErr_enum"
  [VHAL_PTHighPErr_enum] -> UnitConverter104/1
  ZONE_FR_VCU/18(VHAL_PTHighTact_C) -> [VHAL_PTHighTact_C]
  UnitConverter105/1 -> bus_creator/113  "VHAL_PTHighTact_C"
  [VHAL_PTHighTact_C] -> UnitConverter105/1
  ZONE_FR_VCU/19(VHAL_PTHighTactErr_enum) -> [VHAL_PTHighTactErr_enum]
  UnitConverter106/1 -> bus_creator/114  "VHAL_PTHighTactErr_enum"
  [VHAL_PTHighTactErr_enum] -> UnitConverter106/1
  ZONE_FR_VCU/20(VHAL_PTLowP1_KPa) -> [VHAL_PTLowP1_KPa]
  UnitConverter107/1 -> bus_creator/115  "VHAL_PTLowP1_KPa"
  [VHAL_PTLowP1_KPa] -> UnitConverter107/1
  ZONE_FR_VCU/21(VHAL_PTLowP1Err_enum) -> [VHAL_PTLowP1Err_enum]
  UnitConverter108/1 -> bus_creator/116  "VHAL_PTLowP1Err_enum"
  [VHAL_PTLowP1Err_enum] -> UnitConverter108/1
  ZONE_FR_VCU/22(VHAL_PTLowP2_KPa) -> [VHAL_PTLowP2_KPa]
  UnitConverter109/1 -> bus_creator/117  "VHAL_PTLowP2_KPa"
  [VHAL_PTLowP2_KPa] -> UnitConverter109/1
  ZONE_FR_VCU/23(VHAL_PTLowP2Err_enum) -> [VHAL_PTLowP2Err_enum]
  UnitConverter110/1 -> bus_creator/118  "VHAL_PTLowP2Err_enum"
  [VHAL_PTLowP2Err_enum] -> UnitConverter110/1
  ZONE_FR_VCU/24(VHAL_PTLowT1_C) -> [VHAL_PTLowT1_C]
  UnitConverter111/1 -> bus_creator/119  "VHAL_PTLowT1_C"
  [VHAL_PTLowT1_C] -> UnitConverter111/1
  ZONE_FR_VCU/25(VHAL_PTLowT1Err_enum) -> [VHAL_PTLowT1Err_enum]
  UnitConverter112/1 -> bus_creator/120  "VHAL_PTLowT1Err_enum"
  [VHAL_PTLowT1Err_enum] -> UnitConverter112/1
  ZONE_FR_VCU/26(VHAL_PTLowT2_C) -> [VHAL_PTLowT2_C]
  UnitConverter113/1 -> bus_creator/121  "VHAL_PTLowT2_C"
  [VHAL_PTLowT2_C] -> UnitConverter113/1
  ZONE_FR_VCU/27(VHAL_PTLowT2Err_enum) -> [VHAL_PTLowT2Err_enum]
  UnitConverter114/1 -> bus_creator/122  "VHAL_PTLowT2Err_enum"
  [VHAL_PTLowT2Err_enum] -> UnitConverter114/1
  ZONE_FR_VCU/28(VHAL_SOTXVErr_enum) -> [VHAL_SOTXVErr_enum]
  UnitConverter115/1 -> bus_creator/123  "VHAL_SOTXVErr_enum"
  [VHAL_SOTXVErr_enum] -> UnitConverter115/1
  ZONE_FR_VCU/29(VHAL_SOV1Err_enum) -> [VHAL_SOV1Err_enum]
  UnitConverter116/1 -> bus_creator/124  "VHAL_SOV1Err_enum"
  [VHAL_SOV1Err_enum] -> UnitConverter116/1
  ZONE_FR_VCU/30(VHAL_SOV2Err_enum) -> [VHAL_SOV2Err_enum]
  UnitConverter117/1 -> bus_creator/125  "VHAL_SOV2Err_enum"
  [VHAL_SOV2Err_enum] -> UnitConverter117/1
  ZONE_FR_VCU/31(VHAL_SOV3Err_enum) -> [VHAL_SOV3Err_enum]
  UnitConverter118/1 -> bus_creator/126  "VHAL_SOV3Err_enum"
  [VHAL_SOV3Err_enum] -> UnitConverter118/1
  ZONE_FR_VCU/32(VHAL_Tamb_C) -> [VHAL_Tamb_C]
  UnitConverter119/1 -> bus_creator/127  "VHAL_Tamb_C"
  [VHAL_Tamb_C] -> UnitConverter119/1
  ZONE_FR_VCU/33(VHAL_TambErr_enum) -> [VHAL_TambErr_enum]
  UnitConverter120/1 -> bus_creator/128  "VHAL_TambErr_enum"
  [VHAL_TambErr_enum] -> UnitConverter120/1
  VHAL_CANMsgInvalidZONEL1_flg/1(Out) -> bus_creator/129
  ZONE_L1/1(VHAL_ZLDSEATAntiSta_flg) -> [VHAL_ZLDSEATAntiSta_flg]
  UnitConverter121/1 -> bus_creator/130  "VHAL_ZLDSEATAntiSta_flg"
  [VHAL_ZLDSEATAntiSta_flg] -> UnitConverter121/1
  ZONE_L1/2(VHAL_ZLDSEATEntryFunSta_flg) -> [VHAL_ZLDSEATEntryFunSta_flg]
  UnitConverter122/1 -> bus_creator/131  "VHAL_ZLDSEATEntryFunSta_flg"
  [VHAL_ZLDSEATEntryFunSta_flg] -> UnitConverter122/1
  ZONE_L1/3(VHAL_ZLDSEATErrorSta_flg) -> [VHAL_ZLDSEATErrorSta_flg]
  UnitConverter123/1 -> bus_creator/132  "VHAL_ZLDSEATErrorSta_flg"
  [VHAL_ZLDSEATErrorSta_flg] -> UnitConverter123/1
  ZONE_L1/4(VHAL_ZLDSEATMemSetSta_enum) -> [VHAL_ZLDSEATMemSetSta_enum]
  UnitConverter124/1 -> bus_creator/133  "VHAL_ZLDSEATMemSetSta_enum"
  [VHAL_ZLDSEATMemSetSta_enum] -> UnitConverter124/1
  ZONE_L1/5(VHAL_ZLDSEATModeSta_enum) -> [VHAL_ZLDSEATModeSta_enum]
  UnitConverter125/1 -> bus_creator/134  "VHAL_ZLDSEATModeSta_enum"
  [VHAL_ZLDSEATModeSta_enum] -> UnitConverter125/1
  ZONE_L1/6(VHAL_ZLDSEATVentSta_enum) -> [VHAL_ZLDSEATVentSta_enum]
  UnitConverter126/1 -> bus_creator/135  "VHAL_ZLDSEATVentSta_enum"
  [VHAL_ZLDSEATVentSta_enum] -> UnitConverter126/1
  ZONE_L1/7(VHAL_ZLDSEATheaterSta_enum) -> [VHAL_ZLDSEATheaterSta_enum]
  UnitConverter127/1 -> bus_creator/136  "VHAL_ZLDSEATheaterSta_enum"
  [VHAL_ZLDSEATheaterSta_enum] -> UnitConverter127/1
  VHAL_CANMsgInvalidZONEL2_flg/1(Out) -> bus_creator/137
  ZONE_L2/1(VHAL_ZLAPMWinLFOpenedSta_pct) -> [VHAL_ZLAPMWinLFOpenedSta_pct]
  UnitConverter128/1 -> bus_creator/138  "VHAL_ZLAPMWinLFOpenedSta_pct"
  [VHAL_ZLAPMWinLFOpenedSta_pct] -> UnitConverter128/1
  ZONE_L2/2(VHAL_ZLAPMWinLROpenedSta_pct) -> [VHAL_ZLAPMWinLROpenedSta_pct]
  UnitConverter129/1 -> bus_creator/139  "VHAL_ZLAPMWinLROpenedSta_pct"
  [VHAL_ZLAPMWinLROpenedSta_pct] -> UnitConverter129/1
  VHAL_CANMsgInvalidZONER1_flg/1(Out) -> bus_creator/140
  ZONE_R1/1(VHAL_ZRPSEATErrorSta_flg) -> [VHAL_ZRPSEATErrorSta_flg]
  UnitConverter130/1 -> bus_creator/141  "VHAL_ZRPSEATErrorSta_flg"
  [VHAL_ZRPSEATErrorSta_flg] -> UnitConverter130/1
  ZONE_R1/2(VHAL_ZRPSEATModeSta_enum) -> [VHAL_ZRPSEATModeSta_enum]
  UnitConverter131/1 -> bus_creator/142  "VHAL_ZRPSEATModeSta_enum"
  [VHAL_ZRPSEATModeSta_enum] -> UnitConverter131/1
  ZONE_R1/3(VHAL_ZRPSEATVentSta_enum) -> [VHAL_ZRPSEATVentSta_enum]
  UnitConverter132/1 -> bus_creator/143  "VHAL_ZRPSEATVentSta_enum"
  [VHAL_ZRPSEATVentSta_enum] -> UnitConverter132/1
  ZONE_R1/4(VHAL_ZRPSEATheaterSta_enum) -> [VHAL_ZRPSEATheaterSta_enum]
  UnitConverter133/1 -> bus_creator/144  "VHAL_ZRPSEATheaterSta_enum"
  [VHAL_ZRPSEATheaterSta_enum] -> UnitConverter133/1
  ZONE_R1/5(VHAL_ZRPTGActiveSta_enum) -> [VHAL_ZRPTGActiveSta_enum]
  UnitConverter134/1 -> bus_creator/145  "VHAL_ZRPTGActiveSta_enum"
  [VHAL_ZRPTGActiveSta_enum] -> UnitConverter134/1
  ZONE_R1/6(VHAL_ZRPTGExistSta_flg) -> [VHAL_ZRPTGExistSta_flg]
  UnitConverter135/1 -> bus_creator/146  "VHAL_ZRPTGExistSta_flg"
  [VHAL_ZRPTGExistSta_flg] -> UnitConverter135/1
  ZONE_R1/7(VHAL_ZRPTGIsSetHeightSta_flg) -> [VHAL_ZRPTGIsSetHeightSta_flg]
  UnitConverter136/1 -> bus_creator/147  "VHAL_ZRPTGIsSetHeightSta_flg"
  [VHAL_ZRPTGIsSetHeightSta_flg] -> UnitConverter136/1
  ZONE_R1/8(VHAL_ZRPTGSysSta_enum) -> [VHAL_ZRPTGSysSta_enum]
  UnitConverter137/1 -> bus_creator/148  "VHAL_ZRPTGSysSta_enum"
  [VHAL_ZRPTGSysSta_enum] -> UnitConverter137/1
  VHAL_CANMsgInvalidZONER2_flg/1(Out) -> bus_creator/149
  ZONE_R2/1(VHAL_ZRAPMWinRFOpenedSta_pct) -> [VHAL_ZRAPMWinRFOpenedSta_pct]
  UnitConverter138/1 -> bus_creator/150  "VHAL_ZRAPMWinRFOpenedSta_pct"
  [VHAL_ZRAPMWinRFOpenedSta_pct] -> UnitConverter138/1
  ZONE_R2/2(VHAL_ZRAPMWinRROpenedSta_pct) -> [VHAL_ZRAPMWinRROpenedSta_pct]
  UnitConverter139/1 -> bus_creator/151  "VHAL_ZRAPMWinRROpenedSta_pct"
  [VHAL_ZRAPMWinRROpenedSta_pct] -> UnitConverter139/1
  ZONE_R2/3(VHAL_ZRSEATLVentSta_enum) -> [VHAL_ZRSEATLVentSta_enum]
  UnitConverter140/1 -> bus_creator/152  "VHAL_ZRSEATLVentSta_enum"
  [VHAL_ZRSEATLVentSta_enum] -> UnitConverter140/1
  ZONE_R2/4(VHAL_ZRSEATMLVentSta_enum) -> [VHAL_ZRSEATMLVentSta_enum]
  UnitConverter141/1 -> bus_creator/153  "VHAL_ZRSEATMLVentSta_enum"
  [VHAL_ZRSEATMLVentSta_enum] -> UnitConverter141/1
  ZONE_R2/5(VHAL_ZRSEATMRVentSta_enum) -> [VHAL_ZRSEATMRVentSta_enum]
  UnitConverter142/1 -> bus_creator/154  "VHAL_ZRSEATMRVentSta_enum"
  [VHAL_ZRSEATMRVentSta_enum] -> UnitConverter142/1
  ZONE_R2/6(VHAL_ZRSEATRVentSta_enum) -> [VHAL_ZRSEATRVentSta_enum]
  UnitConverter143/1 -> bus_creator/155  "VHAL_ZRSEATRVentSta_enum"
  [VHAL_ZRSEATRVentSta_enum] -> UnitConverter143/1
  VHAL_CANMsgInvalidzGWAPTC1_flg/1(Out) -> bus_creator/156
  zGW_APTC1/1(VHAL_FrntPTCLeActHeatPwr_W) -> [VHAL_FrntPTCLeActHeatPwr_W]
  UnitConverter144/1 -> bus_creator/157  "VHAL_FrntPTCLeActHeatPwr_W"
  [VHAL_FrntPTCLeActHeatPwr_W] -> UnitConverter144/1
  zGW_APTC1/2(VHAL_FrntPTCRearLeActHeatPwr_W) -> [VHAL_FrntPTCRearLeActHeatPwr_W]
  UnitConverter145/1 -> bus_creator/158  "VHAL_FrntPTCRearLeActHeatPwr_W"
  [VHAL_FrntPTCRearLeActHeatPwr_W] -> UnitConverter145/1
  zGW_APTC1/3(VHAL_FrntPTCRearRiActHeatPwr_W) -> [VHAL_FrntPTCRearRiActHeatPwr_W]
  UnitConverter146/1 -> bus_creator/159  "VHAL_FrntPTCRearRiActHeatPwr_W"
  [VHAL_FrntPTCRearRiActHeatPwr_W] -> UnitConverter146/1
  zGW_APTC1/4(VHAL_FrntPTCRiActHeatPwr_W) -> [VHAL_FrntPTCRiActHeatPwr_W]
  UnitConverter147/1 -> bus_creator/160  "VHAL_FrntPTCRiActHeatPwr_W"
  [VHAL_FrntPTCRiActHeatPwr_W] -> UnitConverter147/1
  VHAL_CANMsgInvalidzGWCANFr1_flg/1(Out) -> bus_creator/161
  zGW_CANFr1/1(VHAL_COMPActualPwr_W) -> [VHAL_COMPActualPwr_W]
  UnitConverter148/1 -> bus_creator/162  "VHAL_COMPActualPwr_W"
  [VHAL_COMPActualPwr_W] -> UnitConverter148/1
  zGW_CANFr1/2(VHAL_COMPConCur_A) -> [VHAL_COMPConCur_A]
  UnitConverter149/1 -> bus_creator/163  "VHAL_COMPConCur_A"
  [VHAL_COMPConCur_A] -> UnitConverter149/1
  zGW_CANFr1/3(VHAL_COMPConVolt_V) -> [VHAL_COMPConVolt_V]
  UnitConverter150/1 -> bus_creator/164  "VHAL_COMPConVolt_V"
  [VHAL_COMPConVolt_V] -> UnitConverter150/1
  zGW_CANFr1/4(VHAL_COMPStatorSpd_rpm) -> [VHAL_COMPStatorSpd_rpm]
  UnitConverter151/1 -> bus_creator/165  "VHAL_COMPStatorSpd_rpm"
  [VHAL_COMPStatorSpd_rpm] -> UnitConverter151/1
  zGW_CANFr1/5(VHAL_PTC1PowerConsumption_kW) -> [VHAL_PTC1PowerConsumption_kW]
  UnitConverter152/1 -> bus_creator/166  "VHAL_PTC1PowerConsumption_kW"
  [VHAL_PTC1PowerConsumption_kW] -> UnitConverter152/1
  zGW_CANFr1/6(VHAL_PTCActuPwrHSC6_enum) -> [VHAL_PTCActuPwrHSC6_enum]
  UnitConverter153/1 -> bus_creator/167  "VHAL_PTCActuPwrHSC6_enum"
  [VHAL_PTCActuPwrHSC6_enum] -> UnitConverter153/1
  VHAL_CANMsgInvalidzGWLINDr1_flg/1(Out) -> bus_creator/168
  zGW_LINDr1/1(VHAL_CSWDimSw_flg) -> [VHAL_CSWDimSw_flg]
  UnitConverter154/1 -> bus_creator/169  "VHAL_CSWDimSw_flg"
  [VHAL_CSWDimSw_flg] -> UnitConverter154/1
  zGW_LINDr1/2(VHAL_CSWFWasSwSta_enum) -> [VHAL_CSWFWasSwSta_enum]
  UnitConverter155/1 -> bus_creator/170  "VHAL_CSWFWasSwSta_enum"
  [VHAL_CSWFWasSwSta_enum] -> UnitConverter155/1
  zGW_LINDr1/3(VHAL_CSWFWipSwSta_enum) -> [VHAL_CSWFWipSwSta_enum]
  UnitConverter156/1 -> bus_creator/171  "VHAL_CSWFWipSwSta_enum"
  [VHAL_CSWFWipSwSta_enum] -> UnitConverter156/1
  zGW_LINDr1/4(VHAL_CSWPassSWSta_flg) -> [VHAL_CSWPassSWSta_flg]
  UnitConverter157/1 -> bus_creator/172  "VHAL_CSWPassSWSta_flg"
  [VHAL_CSWPassSWSta_flg] -> UnitConverter157/1
  zGW_LINDr1/5(VHAL_CSWRWasSWSta_enum) -> [VHAL_CSWRWasSWSta_enum]
  UnitConverter158/1 -> bus_creator/173  "VHAL_CSWRWasSWSta_enum"
  [VHAL_CSWRWasSWSta_enum] -> UnitConverter158/1
  zGW_LINDr1/6(VHAL_CSWRWipIntSwSta_enum) -> [VHAL_CSWRWipIntSwSta_enum]
  UnitConverter159/1 -> bus_creator/174  "VHAL_CSWRWipIntSwSta_enum"
  [VHAL_CSWRWipIntSwSta_enum] -> UnitConverter159/1
  zGW_LINDr1/7(VHAL_CSWTurnSwSta_enum) -> [VHAL_CSWTurnSwSta_enum]
  UnitConverter160/1 -> bus_creator/175  "VHAL_CSWTurnSwSta_enum"
  [VHAL_CSWTurnSwSta_enum] -> UnitConverter160/1
  zGW_LINDr1/8(VHAL_FAPWL01LINResponseError_flg) -> [VHAL_FAPWL01LINResponseError_flg]
  UnitConverter161/1 -> bus_creator/176  "VHAL_FAPWL01LINResponseError_flg"
  [VHAL_FAPWL01LINResponseError_flg] -> UnitConverter161/1
  zGW_LINDr1/9(VHAL_LDrvMotorRelayError_flg) -> [VHAL_LDrvMotorRelayError_flg]
  UnitConverter162/1 -> bus_creator/177  "VHAL_LDrvMotorRelayError_flg"
  [VHAL_LDrvMotorRelayError_flg] -> UnitConverter162/1
  zGW_LINDr1/10(VHAL_LDrvMotorRippleError_flg) -> [VHAL_LDrvMotorRippleError_flg]
  UnitConverter163/1 -> bus_creator/178  "VHAL_LDrvMotorRippleError_flg"
  [VHAL_LDrvMotorRippleError_flg] -> UnitConverter163/1
  zGW_LINDr1/11(VHAL_LDrvValWdwOpened_pct) -> [VHAL_LDrvValWdwOpened_pct]
  UnitConverter164/1 -> bus_creator/179  "VHAL_LDrvValWdwOpened_pct"
  [VHAL_LDrvValWdwOpened_pct] -> UnitConverter164/1
  zGW_LINDr1/12(VHAL_LDrvWdwPositionSts_enum) -> [VHAL_LDrvWdwPositionSts_enum]
  UnitConverter165/1 -> bus_creator/180  "VHAL_LDrvWdwPositionSts_enum"
  [VHAL_LDrvWdwPositionSts_enum] -> UnitConverter165/1
  zGW_LINDr1/13(VHAL_LPasMotorRelayError_flg) -> [VHAL_LPasMotorRelayError_flg]
  UnitConverter166/1 -> bus_creator/181  "VHAL_LPasMotorRelayError_flg"
  [VHAL_LPasMotorRelayError_flg] -> UnitConverter166/1
  zGW_LINDr1/14(VHAL_LPasMotorRippleError_flg) -> [VHAL_LPasMotorRippleError_flg]
  UnitConverter167/1 -> bus_creator/182  "VHAL_LPasMotorRippleError_flg"
  [VHAL_LPasMotorRippleError_flg] -> UnitConverter167/1
  zGW_LINDr1/15(VHAL_LPasValWdwOpened_pct) -> [VHAL_LPasValWdwOpened_pct]
  UnitConverter168/1 -> bus_creator/183  "VHAL_LPasValWdwOpened_pct"
  [VHAL_LPasValWdwOpened_pct] -> UnitConverter168/1
  zGW_LINDr1/16(VHAL_LPasWdwPositionSts_enum) -> [VHAL_LPasWdwPositionSts_enum]
  UnitConverter169/1 -> bus_creator/184  "VHAL_LPasWdwPositionSts_enum"
  [VHAL_LPasWdwPositionSts_enum] -> UnitConverter169/1
  zGW_LINDr1/17(VHAL_LRLDMotorRelayError_flg) -> [VHAL_LRLDMotorRelayError_flg]
  UnitConverter170/1 -> bus_creator/185  "VHAL_LRLDMotorRelayError_flg"
  [VHAL_LRLDMotorRelayError_flg] -> UnitConverter170/1
  zGW_LINDr1/18(VHAL_LRLDMotorRippleError_flg) -> [VHAL_LRLDMotorRippleError_flg]
  UnitConverter171/1 -> bus_creator/186  "VHAL_LRLDMotorRippleError_flg"
  [VHAL_LRLDMotorRippleError_flg] -> UnitConverter171/1
  zGW_LINDr1/19(VHAL_LRLDValWdwOpened_pct) -> [VHAL_LRLDValWdwOpened_pct]
  UnitConverter172/1 -> bus_creator/187  "VHAL_LRLDValWdwOpened_pct"
  [VHAL_LRLDValWdwOpened_pct] -> UnitConverter172/1
  zGW_LINDr1/20(VHAL_LRLDWdwPositionSts_enum) -> [VHAL_LRLDWdwPositionSts_enum]
  UnitConverter173/1 -> bus_creator/188  "VHAL_LRLDWdwPositionSts_enum"
  [VHAL_LRLDWdwPositionSts_enum] -> UnitConverter173/1
  zGW_LINDr1/21(VHAL_LRRDMotorRelayError_flg) -> [VHAL_LRRDMotorRelayError_flg]
  UnitConverter174/1 -> bus_creator/189  "VHAL_LRRDMotorRelayError_flg"
  [VHAL_LRRDMotorRelayError_flg] -> UnitConverter174/1
  zGW_LINDr1/22(VHAL_LRRDMotorRippleError_flg) -> [VHAL_LRRDMotorRippleError_flg]
  UnitConverter175/1 -> bus_creator/190  "VHAL_LRRDMotorRippleError_flg"
  [VHAL_LRRDMotorRippleError_flg] -> UnitConverter175/1
  zGW_LINDr1/23(VHAL_LRRDValWdwOpened_pct) -> [VHAL_LRRDValWdwOpened_pct]
  UnitConverter176/1 -> bus_creator/191  "VHAL_LRRDValWdwOpened_pct"
  [VHAL_LRRDValWdwOpened_pct] -> UnitConverter176/1
  zGW_LINDr1/24(VHAL_LRRDWdwPositionSts_enum) -> [VHAL_LRRDWdwPositionSts_enum]
  UnitConverter177/1 -> bus_creator/192  "VHAL_LRRDWdwPositionSts_enum"
  [VHAL_LRRDWdwPositionSts_enum] -> UnitConverter177/1
  zGW_LINDr1/25(VHAL_RAPWL01LINResponseError_flg) -> [VHAL_RAPWL01LINResponseError_flg]
  UnitConverter178/1 -> bus_creator/193  "VHAL_RAPWL01LINResponseError_flg"
  [VHAL_RAPWL01LINResponseError_flg] -> UnitConverter178/1
  zGW_LINDr1/26(VHAL_RLSLampSta_flg) -> [VHAL_RLSLampSta_flg]
  UnitConverter179/1 -> bus_creator/194  "VHAL_RLSLampSta_flg"
  [VHAL_RLSLampSta_flg] -> UnitConverter179/1
  zGW_LINDr1/27(VHAL_RLSRainSnrWiperCmd_enum) -> [VHAL_RLSRainSnrWiperCmd_enum]
  UnitConverter180/1 -> bus_creator/195  "VHAL_RLSRainSnrWiperCmd_enum"
  [VHAL_RLSRainSnrWiperCmd_enum] -> UnitConverter180/1
  zGW_LINDr1/28(VHAL_SWC2LADASSta_flg) -> [VHAL_SWC2LADASSta_flg]
  UnitConverter181/1 -> bus_creator/196  "VHAL_SWC2LADASSta_flg"
  [VHAL_SWC2LADASSta_flg] -> UnitConverter181/1
  zGW_LINDr1/29(VHAL_SWC2LDriveModeSta_flg) -> [VHAL_SWC2LDriveModeSta_flg]
  UnitConverter182/1 -> bus_creator/197  "VHAL_SWC2LDriveModeSta_flg"
  [VHAL_SWC2LDriveModeSta_flg] -> UnitConverter182/1
  zGW_LINDr1/30(VHAL_SWC2LHomeSta_flg) -> [VHAL_SWC2LHomeSta_flg]
  UnitConverter183/1 -> bus_creator/198  "VHAL_SWC2LHomeSta_flg"
  [VHAL_SWC2LHomeSta_flg] -> UnitConverter183/1
  zGW_LINDr1/31(VHAL_SWC2LLeftSta_flg) -> [VHAL_SWC2LLeftSta_flg]
  UnitConverter184/1 -> bus_creator/199  "VHAL_SWC2LLeftSta_flg"
  [VHAL_SWC2LLeftSta_flg] -> UnitConverter184/1
  zGW_LINDr1/32(VHAL_SWC2LRightSta_flg) -> [VHAL_SWC2LRightSta_flg]
  UnitConverter185/1 -> bus_creator/200  "VHAL_SWC2LRightSta_flg"
  [VHAL_SWC2LRightSta_flg] -> UnitConverter185/1
  zGW_LINDr1/33(VHAL_SWC2LScrollDownSta_flg) -> [VHAL_SWC2LScrollDownSta_flg]
  UnitConverter186/1 -> bus_creator/201  "VHAL_SWC2LScrollDownSta_flg"
  [VHAL_SWC2LScrollDownSta_flg] -> UnitConverter186/1
  zGW_LINDr1/34(VHAL_SWC2LScrollPressSta_flg) -> [VHAL_SWC2LScrollPressSta_flg]
  UnitConverter187/1 -> bus_creator/202  "VHAL_SWC2LScrollPressSta_flg"
  [VHAL_SWC2LScrollPressSta_flg] -> UnitConverter187/1
  zGW_LINDr1/35(VHAL_SWC2LScrollUpSta_flg) -> [VHAL_SWC2LScrollUpSta_flg]
  UnitConverter188/1 -> bus_creator/203  "VHAL_SWC2LScrollUpSta_flg"
  [VHAL_SWC2LScrollUpSta_flg] -> UnitConverter188/1
  zGW_LINDr1/36(VHAL_SWC2RCustomizeSta_flg) -> [VHAL_SWC2RCustomizeSta_flg]
  UnitConverter189/1 -> bus_creator/204  "VHAL_SWC2RCustomizeSta_flg"
  [VHAL_SWC2RCustomizeSta_flg] -> UnitConverter189/1
  zGW_LINDr1/37(VHAL_SWC2RLeftSta_flg) -> [VHAL_SWC2RLeftSta_flg]
  UnitConverter190/1 -> bus_creator/205  "VHAL_SWC2RLeftSta_flg"
  [VHAL_SWC2RLeftSta_flg] -> UnitConverter190/1
  zGW_LINDr1/38(VHAL_SWC2RPageSwitchSta_flg) -> [VHAL_SWC2RPageSwitchSta_flg]
  UnitConverter191/1 -> bus_creator/206  "VHAL_SWC2RPageSwitchSta_flg"
  [VHAL_SWC2RPageSwitchSta_flg] -> UnitConverter191/1
  zGW_LINDr1/39(VHAL_SWC2RRightSta_flg) -> [VHAL_SWC2RRightSta_flg]
  UnitConverter192/1 -> bus_creator/207  "VHAL_SWC2RRightSta_flg"
  [VHAL_SWC2RRightSta_flg] -> UnitConverter192/1
  zGW_LINDr1/40(VHAL_SWC2RScrollDownSta_flg) -> [VHAL_SWC2RScrollDownSta_flg]
  UnitConverter193/1 -> bus_creator/208  "VHAL_SWC2RScrollDownSta_flg"
  [VHAL_SWC2RScrollDownSta_flg] -> UnitConverter193/1
  zGW_LINDr1/41(VHAL_SWC2RScrollPressSta_flg) -> [VHAL_SWC2RScrollPressSta_flg]
  UnitConverter194/1 -> bus_creator/209  "VHAL_SWC2RScrollPressSta_flg"
  [VHAL_SWC2RScrollPressSta_flg] -> UnitConverter194/1
  zGW_LINDr1/42(VHAL_SWC2RScrollUpSta_flg) -> [VHAL_SWC2RScrollUpSta_flg]
  UnitConverter195/1 -> bus_creator/210  "VHAL_SWC2RScrollUpSta_flg"
  [VHAL_SWC2RScrollUpSta_flg] -> UnitConverter195/1
  zGW_LINDr1/43(VHAL_SWC2RVRSta_flg) -> [VHAL_SWC2RVRSta_flg]
  UnitConverter196/1 -> bus_creator/211  "VHAL_SWC2RVRSta_flg"
  [VHAL_SWC2RVRSta_flg] -> UnitConverter196/1
  zGW_LINDr1/44(VHAL_SWCACCSta_flg) -> [VHAL_SWCACCSta_flg]
  UnitConverter197/1 -> bus_creator/212  "VHAL_SWCACCSta_flg"
  [VHAL_SWCACCSta_flg] -> UnitConverter197/1
  zGW_LINDr1/45(VHAL_SWCCANCELSta_flg) -> [VHAL_SWCCANCELSta_flg]
  UnitConverter198/1 -> bus_creator/213  "VHAL_SWCCANCELSta_flg"
  [VHAL_SWCCANCELSta_flg] -> UnitConverter198/1
  zGW_LINDr1/46(VHAL_SWCDistanceSta_flg) -> [VHAL_SWCDistanceSta_flg]
  UnitConverter199/1 -> bus_creator/214  "VHAL_SWCDistanceSta_flg"
  [VHAL_SWCDistanceSta_flg] -> UnitConverter199/1
  zGW_LINDr1/47(VHAL_SWCDownSta_flg) -> [VHAL_SWCDownSta_flg]
  UnitConverter200/1 -> bus_creator/215  "VHAL_SWCDownSta_flg"
  [VHAL_SWCDownSta_flg] -> UnitConverter200/1
  zGW_LINDr1/48(VHAL_SWCLKASta_flg) -> [VHAL_SWCLKASta_flg]
  UnitConverter201/1 -> bus_creator/216  "VHAL_SWCLKASta_flg"
  [VHAL_SWCLKASta_flg] -> UnitConverter201/1
  zGW_LINDr1/49(VHAL_SWCLeftSta_flg) -> [VHAL_SWCLeftSta_flg]
  UnitConverter202/1 -> bus_creator/217  "VHAL_SWCLeftSta_flg"
  [VHAL_SWCLeftSta_flg] -> UnitConverter202/1
  zGW_LINDr1/50(VHAL_SWCRegenDown_flg) -> [VHAL_SWCRegenDown_flg]
  UnitConverter203/1 -> bus_creator/218  "VHAL_SWCRegenDown_flg"
  [VHAL_SWCRegenDown_flg] -> UnitConverter203/1
  zGW_LINDr1/51(VHAL_SWCRegenUp_flg) -> [VHAL_SWCRegenUp_flg]
  UnitConverter204/1 -> bus_creator/219  "VHAL_SWCRegenUp_flg"
  [VHAL_SWCRegenUp_flg] -> UnitConverter204/1
  zGW_LINDr1/52(VHAL_SWCResUpSta_flg) -> [VHAL_SWCResUpSta_flg]
  UnitConverter205/1 -> bus_creator/220  "VHAL_SWCResUpSta_flg"
  [VHAL_SWCResUpSta_flg] -> UnitConverter205/1
  zGW_LINDr1/53(VHAL_SWCRightSta_flg) -> [VHAL_SWCRightSta_flg]
  UnitConverter206/1 -> bus_creator/221  "VHAL_SWCRightSta_flg"
  [VHAL_SWCRightSta_flg] -> UnitConverter206/1
  zGW_LINDr1/54(VHAL_SWCSetdownSta_flg) -> [VHAL_SWCSetdownSta_flg]
  UnitConverter207/1 -> bus_creator/222  "VHAL_SWCSetdownSta_flg"
  [VHAL_SWCSetdownSta_flg] -> UnitConverter207/1
  zGW_LINDr1/55(VHAL_SWCTripSta_flg) -> [VHAL_SWCTripSta_flg]
  UnitConverter208/1 -> bus_creator/223  "VHAL_SWCTripSta_flg"
  [VHAL_SWCTripSta_flg] -> UnitConverter208/1
  zGW_LINDr1/56(VHAL_SWCUndefinedSta_flg) -> [VHAL_SWCUndefinedSta_flg]
  UnitConverter209/1 -> bus_creator/224  "VHAL_SWCUndefinedSta_flg"
  [VHAL_SWCUndefinedSta_flg] -> UnitConverter209/1
  zGW_LINDr1/57(VHAL_SWCUpSta_flg) -> [VHAL_SWCUpSta_flg]
  UnitConverter210/1 -> bus_creator/225  "VHAL_SWCUpSta_flg"
  [VHAL_SWCUpSta_flg] -> UnitConverter210/1
  zGW_LINDr1/58(VHAL_SWCVRSta_flg) -> [VHAL_SWCVRSta_flg]
  UnitConverter211/1 -> bus_creator/226  "VHAL_SWCVRSta_flg"
  [VHAL_SWCVRSta_flg] -> UnitConverter211/1
  zGW_LINDr1/59(VHAL_SWCmodeSta_flg) -> [VHAL_SWCmodeSta_flg]
  UnitConverter212/1 -> bus_creator/227  "VHAL_SWCmodeSta_flg"
  [VHAL_SWCmodeSta_flg] -> UnitConverter212/1
  VHAL_CANMsgInvalidzGWLINFr1_flg/1(Out) -> bus_creator/228
  zGW_LINFr1/1(VHAL_AGSActualPosition_enum) -> [VHAL_AGSActualPosition_enum]
  UnitConverter213/1 -> bus_creator/229  "VHAL_AGSActualPosition_enum"
  [VHAL_AGSActualPosition_enum] -> UnitConverter213/1
  VHAL_CANMsgInvalidzGWSEAT1_flg/1(Out) -> bus_creator/230
  zGW_SEAT1/1(VHAL_DSEATAntiSta_flg) -> [VHAL_DSEATAntiSta_flg]
  UnitConverter214/1 -> bus_creator/231  "VHAL_DSEATAntiSta_flg"
  [VHAL_DSEATAntiSta_flg] -> UnitConverter214/1
  zGW_SEAT1/2(VHAL_DSEATEntryFunSta_flg) -> [VHAL_DSEATEntryFunSta_flg]
  UnitConverter215/1 -> bus_creator/232  "VHAL_DSEATEntryFunSta_flg"
  [VHAL_DSEATEntryFunSta_flg] -> UnitConverter215/1
  zGW_SEAT1/3(VHAL_DSEATErrorSta_flg) -> [VHAL_DSEATErrorSta_flg]
  UnitConverter216/1 -> bus_creator/233  "VHAL_DSEATErrorSta_flg"
  [VHAL_DSEATErrorSta_flg] -> UnitConverter216/1
  zGW_SEAT1/4(VHAL_DSEATHWVer_enum) -> [VHAL_DSEATHWVer_enum]
  UnitConverter217/1 -> bus_creator/234  "VHAL_DSEATHWVer_enum"
  [VHAL_DSEATHWVer_enum] -> UnitConverter217/1
  zGW_SEAT1/5(VHAL_DSEATMode_enum) -> [VHAL_DSEATMode_enum]
  UnitConverter218/1 -> bus_creator/235  "VHAL_DSEATMode_enum"
  [VHAL_DSEATMode_enum] -> UnitConverter218/1
  zGW_SEAT1/6(VHAL_DSEATSWVer_enum) -> [VHAL_DSEATSWVer_enum]
  UnitConverter219/1 -> bus_creator/236  "VHAL_DSEATSWVer_enum"
  [VHAL_DSEATSWVer_enum] -> UnitConverter219/1
  zGW_SEAT1/7(VHAL_DSEATVentSta_enum) -> [VHAL_DSEATVentSta_enum]
  UnitConverter220/1 -> bus_creator/237  "VHAL_DSEATVentSta_enum"
  [VHAL_DSEATVentSta_enum] -> UnitConverter220/1
  zGW_SEAT1/8(VHAL_DSEATheatersta_enum) -> [VHAL_DSEATheatersta_enum]
  UnitConverter221/1 -> bus_creator/238  "VHAL_DSEATheatersta_enum"
  [VHAL_DSEATheatersta_enum] -> UnitConverter221/1
  zGW_SEAT1/9(VHAL_PSEATErrorSta_flg) -> [VHAL_PSEATErrorSta_flg]
  UnitConverter222/1 -> bus_creator/239  "VHAL_PSEATErrorSta_flg"
  [VHAL_PSEATErrorSta_flg] -> UnitConverter222/1
  zGW_SEAT1/10(VHAL_PSEATHWVer_enum) -> [VHAL_PSEATHWVer_enum]
  UnitConverter223/1 -> bus_creator/240  "VHAL_PSEATHWVer_enum"
  [VHAL_PSEATHWVer_enum] -> UnitConverter223/1
  zGW_SEAT1/11(VHAL_PSEATMode_enum) -> [VHAL_PSEATMode_enum]
  UnitConverter224/1 -> bus_creator/241  "VHAL_PSEATMode_enum"
  [VHAL_PSEATMode_enum] -> UnitConverter224/1
  zGW_SEAT1/12(VHAL_PSEATSWVer_enum) -> [VHAL_PSEATSWVer_enum]
  UnitConverter225/1 -> bus_creator/242  "VHAL_PSEATSWVer_enum"
  [VHAL_PSEATSWVer_enum] -> UnitConverter225/1
  zGW_SEAT1/13(VHAL_PSEATVentSta_enum) -> [VHAL_PSEATVentSta_enum]
  UnitConverter226/1 -> bus_creator/243  "VHAL_PSEATVentSta_enum"
  [VHAL_PSEATVentSta_enum] -> UnitConverter226/1
  zGW_SEAT1/14(VHAL_PSEATheatersta_enum) -> [VHAL_PSEATheatersta_enum]
  UnitConverter227/1 -> bus_creator/244  "VHAL_PSEATheatersta_enum"
  [VHAL_PSEATheatersta_enum] -> UnitConverter227/1
